simulink model "R2RSystemModel_no_state_filter"  (R2014a)
settings: Solver=ode45  StartTime=StartTime  StopTime=StopTime  MaxStep=MaxStepSize  RelTol=1e-3
values from neighbouring files (symbols this model uses):
  K_L12_Force = 2.29181    [ControlDesign.m]    (also in ControlDesignForceModeLinear.m)
  K_PWM = PWM_res/V_rail    (= 83.3333333333)    [ControlDesign.m]    (also in ControlDesignForceModeLinear.m = 0.012)
  Kspring = 55    [ControlDesign.m]    (also in ControlDesignForceModeLinear.m = 100)
  L12_Offset_I = 12.995    [ControlDesign.m]    (also in ControlDesignForceModeLinear.m)
  PWM_res = 2000    [ControlDesign.m]    (also in ControlDesignForceModeLinear.m)
  Ra_L12 = 60    [ControlDesign.m]    (also in ControlDesignForceModeLinear.m)
libraries: simulink x1
settings Model: Creator=oberstare  LastModifiedBy=oberstare

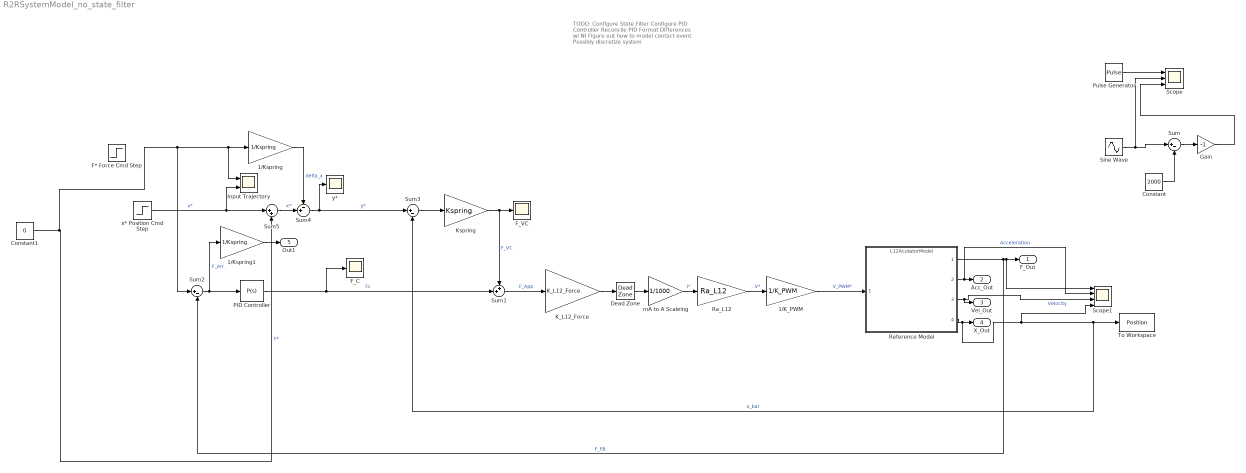
== system R2RSystemModel_no_state_filter ==
  note: TODO:
      | Configure State Filter
      | Configure PID Controller
      | Reconcile PID Format Differences w/ NI
      | Figure out how to model contact event
      | Possibly discretize system
  1/K_PWM : Gain  Gain=1/K_PWM
  1/Kspring : Gain  Gain=1/Kspring
  1/Kspring1 : Gain  Gain=1/Kspring
  Constant : Constant  Value=2000
  Constant1 : Constant  Value=0
  Dead Zone : DeadZone  LowerValue=-1000/L12_Offset_I  UpperValue=1000/L12_Offset_I  SaturateOnIntegerOverflow=on
  F* Force Cmd Step : Step  Time=60  SampleTime=0
  F_C : Scope
      settings: SaveName=ScopeData2
  F_VC : Scope
  Gain : Gain  Gain=-1
  "Input Trajectory " : Scope  NumInputPorts=2
      settings: YMin=-5~-5  YMax=5~5  SaveName=ScopeData3
  K_L12_Force : Gain  Gain=K_L12_Force
  Kspring : Gain  Gain=Kspring
  PID Controller : simulink/Continuous/PID Controller  Controller=P  TimeDomain=Continuous-time  SampleTime=1  IntegratorMethod=Forward Euler  FilterMethod=Forward Euler  Form=Parallel  P=0  I=1  D=0  N=100  InitialConditionSource=internal  InitialConditionForIntegrator=0  InitialConditionForFilter=0  ExternalReset=none  LimitOutput=off  UpperSaturationLimit=inf  LowerSaturationLimit=-inf  LinearizeAsGain=on  AntiWindupMode=none  Kb=1  TrackingMode=off  Kt=1  PParamMin=[]  PParamMax=[]  IParamMin=[]  IParamMax=[]  DParamMin=[]  DParamMax=[]  NParamMin=[]  NParamMax=[]  KbParamMin=[]  KbParamMax=[]  KtParamMin=[]  KtParamMax=[]  POutMin=[]  POutMax=[]  IOutMin=[]  IOutMax=[]  DOutMin=[]  DOutMax=[]  NOutMin=[]  NOutMax=[]  KbOutMin=[]  KbOutMax=[]  KtOutMin=[]  KtOutMax=[]  IntegratorOutMin=[]  IntegratorOutMax=[]  FilterOutMin=[]  FilterOutMax=[]  SumOutMin=[]  SumOutMax=[]  SumI1OutMin=[]  SumI1OutMax=[]  SumI2OutMin=[]  SumI2OutMax=[]  SumI3OutMin=[]  SumI3OutMax=[]  SumDOutMin=[]  SumDOutMax=[]  SaturationOutMin=[]  SaturationOutMax=[]  IntegratorContinuousStateAttributes=''  IntegratorStateMustResolveToSignalObject=off  IntegratorRTWStateStorageClass=Auto  FilterContinuousStateAttributes=''  FilterStateMustResolveToSignalObject=off  FilterRTWStateStorageClass=Auto
  Pulse Generator : DiscretePulseGenerator  PulseType=Time based  Amplitude=4000  Period=10  PulseWidth=50  PhaseDelay=2.5
  Ra_L12 : Gain  Gain=Ra_L12
  Reference Model : ModelReference  ModelNameDialog=L12AcutatorModel.slx  SimulationMode=Normal  ModelReferenceVersion=1.20  CopyOfModelName=L12AcutatorModel.slx  DefaultDataLogging=on
  Scope : Scope  NumInputPorts=3
      settings: YMin=-5~-5~-5  YMax=5~5~5  SaveName=ScopeData7
  Scope1 : Scope  NumInputPorts=4
      settings: YMin=-5~-5~-5~-5  YMax=5~5~5~5  SaveName=ScopeData4
  Sine Wave : Sin  Amplitude=PWM_res  Bias=PWM_res  Phase=pi/2  SampleTime=0
  Sum : Sum  Inputs=|+-
  Sum1 : Sum  Inputs=++|
  Sum2 : Sum  Inputs=|+-
  Sum3 : Sum  Inputs=|+-
  Sum4 : Sum  Inputs=-+|
  Sum5 : Sum  Inputs=|++
  To Workspace : ToWorkspace  VariableName=Position  SaveFormat=Timeseries  SampleTime=-1
  mA to A Scaleing : Gain  Gain=1/1000
  x* Position Cmd Step : Step  Time=5  After=30  SampleTime=0
  y* : Scope
  F_Out : Outport
  Acc_Out : Outport  Port=2
  Vel_Out : Outport  Port=3
  X_Out : Outport  Port=4
  Out1 : Outport  Port=5
  wires:
  Reference Model/1 -> Scope1/1, F_Out/1, Sum2/2  "F_FB"
  Reference Model/2 -> Scope1/2, Acc_Out/1  "Acceleration"
  Reference Model/3 -> Scope1/3, Vel_Out/1  "Velocity"
  Constant/1 -> Sum/2
  Sum/1 -> Gain/1
  Gain/1 -> Scope/3
  Sine Wave/1 -> Scope/2, Sum/1
  Pulse Generator/1 -> Scope/1
  Reference Model/4 -> Scope1/4, Sum3/2, To Workspace/1, X_Out/1  "x_bar"
  Ra_L12/1 -> 1/K_PWM/1  "V*"
  1/K_PWM/1 -> Reference Model/1  "V_PWM*"
  mA to A Scaleing/1 -> Ra_L12/1  "I*"
  Dead Zone/1 -> mA to A Scaleing/1
  K_L12_Force/1 -> Dead Zone/1
  Sum1/1 -> K_L12_Force/1  "F_App"
  Kspring/1 -> F_VC/1, Sum1/1  "F_VC"
  Sum3/1 -> Kspring/1
  Constant1/1 -> "Input Trajectory "/1, 1/Kspring/1, Sum2/1, Sum5/2  "F*"
  1/Kspring/1 -> Sum4/1  "delta_x"
  Sum2/1 -> PID Controller/1, 1/Kspring1/1  "F_err"
  PID Controller/1 -> F_C/1, Sum1/2  "Fc"
  x* Position Cmd Step/1 -> "Input Trajectory "/2, Sum5/1  "x*"
  Sum5/1 -> Sum4/2  "x*'"
  Sum4/1 -> Sum3/1, y*/1  "y*"
  1/Kspring1/1 -> Out1/1
